simulink model "stellaris_lp_irreceive_NEC"  (R2017a)
settings: Solver=FixedStepDiscrete  StartTime=0.0  StopTime=0.5  FixedStep=ts  RelTol=1e-3  EnableMultiTasking=on
undefined symbols (not defined in the file or in its folder): ts
libraries: simulink x5, stellaris_lp_lib x4
settings Model: ExtModeTrigDuration=2  Creator=peselnikmg  LastModifiedBy=Nilim
settings DataIOCC: LimitDataPoints=on  SaveFormat=Array  SignalLoggingSaveFormat=ModelDataLogs  ReturnWorkspaceOutputs=on
settings OptimizationCC: UseDivisionForNetSlopeComputation=on  UseFloatMulNetSlope=on  UseSpecifiedMinMax=on  PassReuseOutputArgsAs=Individual arguments  ExpressionDepthLimit=2147483647  ZeroExternalMemoryAtStartup=off  ZeroInternalMemoryAtStartup=off  NoFixptDivByZeroProtection=on  EfficientFloat2IntCast=on  LifeSpan=inf  MaxStackSize=64  OptimizeBlockOrder=speed
settings DebuggingCC: ReadBeforeWriteMsg=DisableAll  WriteAfterWriteMsg=DisableAll  WriteAfterReadMsg=DisableAll  MultiTaskDSMMsg=none  IntegerOverflowMsg=error  ParameterTunabilityLossMsg=error  AssertControl=DisableAll  StateNameClashWarn=warning  NonBusSignalsTreatedAsBus=error  SFInvalidInputDataAccessInChartInitDiag=error  SFTransitionOutsideNaturalParentDiag=error  SFUnreachableExecutionPathDiag=error  SFUndirectedBroadcastEventsDiag=error  SFExecutionAtInitializationDiag=none  IntegerSaturationMsg=error
settings HardwareCC: ProdBitPerPointer=32  ProdBitPerSizeT=32  ProdBitPerPtrDiffT=32  ProdLargestAtomicInteger=Long  ProdLargestAtomicFloat=Double  ProdWordSize=32  ProdHWDeviceType=ARM Compatible->ARM Cortex
settings ModelReferenceCC: UpdateModelReferenceTargets=IfOutOfDate  PropagateSignalLabelsOutOfModel=off
settings SFSimCC: SFSimEcho=off  MATLABDynamicMemAlloc=off
settings RTWCC: SystemTargetFile=ert.tlc  HardwareBoard=Tiva TM4C123G Launchpad  TLCOptions=-aInlineSetEventsForThisBaseRateFcn=TLC_FALSE -aSuppressMultiTaskScheduler=TLC_FALSE -aRateBasedStepFcn=1  TemplateMakefile=ert_default_tmf  Description=Embedded Coder  GenerateReport=on  RTWVerbose=off  Toolchain=Texas Instruments Code Composer Studio (Tiva)  BuildConfiguration=Faster Runs  IncludeHyperlinkInReport=on  LaunchReport=on  GenerateTraceInfo=on  GenerateTraceReport=on  GenerateTraceReportSl=on  GenerateTraceReportSf=on  GenerateTraceReportEml=on
settings CodeAppCC: ForceParamTrailComments=on  IgnoreCustomStorageClasses=off  OperatorAnnotations=on  SimulinkDataObjDesc=on  SFDataObjDesc=on  MATLABFcnDesc=on  CustomSymbolStrType=$N$R$M  InsertBlockDesc=on  MATLABSourceComments=on  EnableCustomComments=on  ReqsInCode=on
settings ERTTargetCC: UtilityFuncGeneration=Shared location  CombineSignalStateStructs=on  SuppressErrorStatus=on  SupportNonFinite=off  ParenthesesLevel=Maximum  CastingMode=Standards  EnableSignedLeftShifts=off  EnableSignedRightShifts=off
settings ConfigComp: CovMetricSettings=dw  CovHtmlReporting=on  CovSaveCumulativeToWorkspaceVar=on  CovSaveSingleToWorkspaceVar=on  CovExternalEMLEnable=off

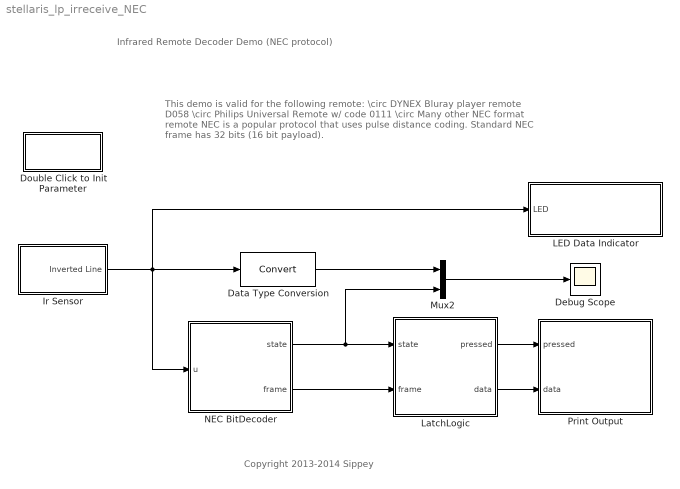
== system stellaris_lp_irreceive_NEC ==
  note: This demo is valid for the following remote:
      | \circ  DYNEX Bluray player remote D058
      | \circ  Philips Universal Remote w/ code 0111
      | \circ  Many other NEC format remote
      |
      | NEC is a popular protocol that uses pulse distance coding. Standard
      | NEC frame has 32 bits (16 bit payload).
  note: Infrared Remote Decoder Demo (NEC protocol)
  note: Copyright 2013-2014 Sippey
  Data Type Conversion : DataTypeConversion  SampleTime=ts
  Debug Scope : Scope
  Double Click to Init Parameter : Subsystem
      settings: OpenFcn=ts=0.0001;
      mask Display: fprintf('Double-click');
  Ir Sensor : Subsystem
  LED Data Indicator : Subsystem
  LatchLogic : Stateflow chart  TreatAsAtomicUnit=on
  Mux2 : Mux  Inputs=2
  NEC BitDecoder : Stateflow chart  TreatAsAtomicUnit=on
  Print Output : Subsystem
  wires:
  Mux2/1 -> Debug Scope/1
  Ir Sensor/1(Inverted Line) -> NEC BitDecoder/1(u), Data Type Conversion/1, LED Data Indicator/1(LED)
  NEC BitDecoder/1(state) -> LatchLogic/1(state), Mux2/2
  Data Type Conversion/1 -> Mux2/1
  NEC BitDecoder/2(frame) -> LatchLogic/2(frame)
  LatchLogic/1(pressed) -> Print Output/1(pressed)
  LatchLogic/2(data) -> Print Output/2(data)

== system stellaris_lp_irreceive_NEC/Double Click to Init Parameter ==

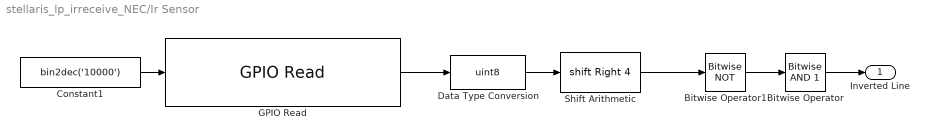
== system stellaris_lp_irreceive_NEC/Ir Sensor ==
  Bitwise Operator : simulink/Logic and Bit Operations/Bitwise Operator  logicop=AND  UseBitMask=on  BitMask=1  BitMaskRealWorld=Stored Integer
  Bitwise Operator1 : simulink/Logic and Bit Operations/Bitwise Operator  logicop=NOT  UseBitMask=off  BitMask=1  BitMaskRealWorld=Stored Integer
  Constant1 : Constant  Value=bin2dec('10000')  OutDataTypeStr=Inherit: Inherit via back propagation
  Data Type Conversion : DataTypeConversion  OutDataTypeStr=uint8  SampleTime=ts
  GPIO Read : stellaris_lp_lib/GPIO/GPIO Read  GPIO_PORTX_BASE=GPIO_PORTF_BASE  SampleTime=-1
      settings: SourceProductName=Run on Stellaris LaunchPad
  Shift Arithmetic : ArithShift  BitShiftNumber=4  BitShiftDirection=Right
  Inverted Line : Outport
  wires:
  Constant1/1 -> GPIO Read/1
  Shift Arithmetic/1 -> Bitwise Operator1/1
  GPIO Read/1 -> Data Type Conversion/1
  Bitwise Operator1/1 -> Bitwise Operator/1
  Bitwise Operator/1 -> Inverted Line/1
  Data Type Conversion/1 -> Shift Arithmetic/1

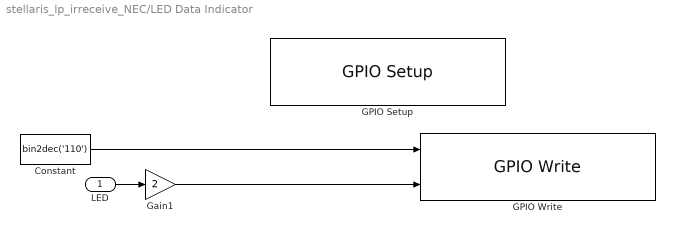
== system stellaris_lp_irreceive_NEC/LED Data Indicator ==
  LED : Inport
  Constant : Constant  Value=bin2dec('110')  OutDataTypeStr=Inherit: Inherit via back propagation
  GPIO Setup : stellaris_lp_lib/GPIO/GPIO Setup  GPIO_PORTX_BASE=GPIO_PORTF_BASE  PinsOutput_0=Input  PinsOutput_1=Output  PinsOutput_2=Output  PinsOutput_3=Output  PinsOutput_4=Input  PinsOutput_5=Input  PinsOutput_6=Input  PinsOutput_7=Input
      settings: SourceProductName=Run on Stellaris LaunchPad
  GPIO Write : stellaris_lp_lib/GPIO/GPIO Write  GPIO_PORTX_BASE=GPIO_PORTF_BASE  SampleTime=-1
      settings: SourceProductName=Run on Stellaris LaunchPad
  Gain1 : Gain  Gain=2  OutDataTypeStr=Inherit: Inherit via back propagation
  wires:
  Constant/1 -> GPIO Write/1
  Gain1/1 -> GPIO Write/2
  LED/1 -> Gain1/1

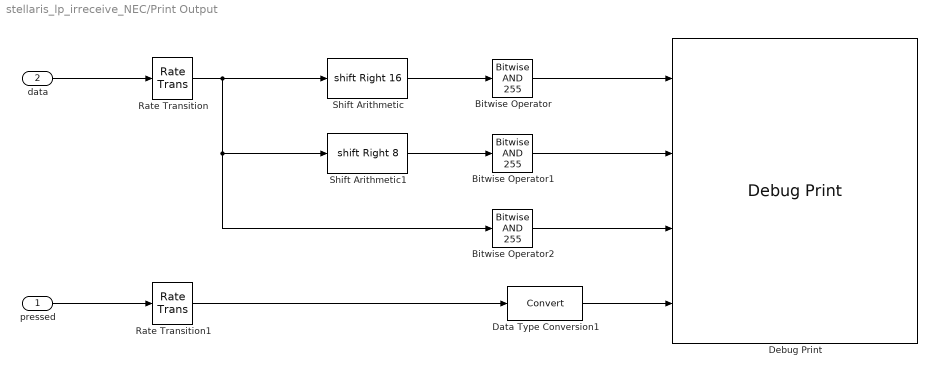
== system stellaris_lp_irreceive_NEC/Print Output ==
  pressed : Inport
  data : Inport  Port=2
  Bitwise Operator : simulink/Logic and Bit Operations/Bitwise Operator  logicop=AND  UseBitMask=on  BitMask=255  BitMaskRealWorld=Stored Integer
  Bitwise Operator1 : simulink/Logic and Bit Operations/Bitwise Operator  logicop=AND  UseBitMask=on  BitMask=255  BitMaskRealWorld=Stored Integer
  Bitwise Operator2 : simulink/Logic and Bit Operations/Bitwise Operator  logicop=AND  UseBitMask=on  BitMask=255  BitMaskRealWorld=Stored Integer
  Data Type Conversion1 : DataTypeConversion
  Debug Print : stellaris_lp_lib/Debug/Debug Print  fmt='addr1: %02X, addr2: %02X, key %d, pressed %d'  sample_time=0.1
      settings: SourceProductName=Run on Stellaris LaunchPad
  Rate Transition : RateTransition
  Rate Transition1 : RateTransition
  Shift Arithmetic : ArithShift  BitShiftNumber=16  BitShiftDirection=Right
  Shift Arithmetic1 : ArithShift  BitShiftNumber=8  BitShiftDirection=Right
  wires:
  Shift Arithmetic/1 -> Bitwise Operator/1
  Bitwise Operator/1 -> Debug Print/1
  Shift Arithmetic1/1 -> Bitwise Operator1/1
  Rate Transition/1 -> Bitwise Operator2/1, Shift Arithmetic1/1, Shift Arithmetic/1
  Bitwise Operator1/1 -> Debug Print/2
  Bitwise Operator2/1 -> Debug Print/3
  Rate Transition1/1 -> Data Type Conversion1/1
  data/1 -> Rate Transition/1
  Data Type Conversion1/1 -> Debug Print/4
  pressed/1 -> Rate Transition1/1

== stateflow chart stellaris_lp_irreceive_NEC/LatchLogic ==
  state NotPressed
    pressed=0;
    data=0;
  state Pressed
    pressed=1;
  note: If repeat stub is seen, the bit decoder will go
      | to the BitDecoded state once and then timeout.
      | Reset the temporal logic at this time.
  note: timeout after 125ms
      | if a repeat stub have
      | not show up yet
  (default) -> NotPressed
  NotPressed -> Pressed : [state==1]{data=frame;}
  Pressed -> Pressed [order 2] : [state==-4]
  Pressed -> NotPressed [order 1] : after(0.125,sec)
  data: state input int32 =0; frame input int32; pressed output int32; data output int32

== stateflow chart stellaris_lp_irreceive_NEC/NEC BitDecoder ==
  note: bit detection timeout 10ms
  note: bit '0': 562.5µs space
      | bit '1': 1.6875ms  space
      | Threshold set to 1ms
  note: invalid start bit
  note: 9ms start pulse
      | set 8ms as threshold
  state StartSym
    state = -2;
  state BitWait
    state= -3;
  state Idle
    state = -1;
    frame=0;
  state BitDecoded
    state=-4;
  state OutStage
    state=1;
  note: output trigger
      | valid for one tick
  note: space between start bit and first data
      | pulse is 4.5ms and will be decoded
      | as a '1' bit, so one more bit to decode.
  BitWait -> Idle [order 3] : after(10e-3,sec)
  (default) -> Idle
  StartSym -> BitWait [order 1] : after(8e-3,sec)
      | [u==0]
      | {nb=0;frame=0;}
  StartSym -> Idle [order 2] : before(8e-3,sec)[u==0]
  BitWait -> BitDecoded [order 2] : after(1e-3,sec)[u==1]{frame=2*frame+1;}
  BitWait -> BitDecoded [order 4] : before(1e-3,sec)[u==1]{frame=2*frame;}
  Idle -> StartSym : [u==1]
  BitDecoded -> BitWait : [u==0]{nb=nb+1;}
  OutStage -> Idle
  BitWait -> OutStage [order 1] : [nb>=25]
  data: u input; state output int32 =0; nb local int32; frame output int32
